simulink model "lidar_obstacle"  (R2020b)
settings: Solver=VariableStepAuto  StartTime=0.0  StopTime=Tf  RelTol=1e-3
values from neighbouring files (symbols this model uses):
  maze = imcomplement(maze)    [Run_Sim_LC.m]
  N = size(waypoints, 1)    [interpolate_leg_waypoints.m]
  startPose = [2 2 0]    [Run_Sim_LC.m]
  Ts = 0.01    [Run_Sim_LC.m]
  x = k4*t^4 + k3*t^3 + k2*t^2 + k1*t + k0    [get_leg_waypoints_symb.m]    (also in leg_ik_symb.m = r*cos(phi); leg_ik_symb_hexa.m = r*cos(phi+alpha))
  y = r*sin(phi)    [leg_ik_symb.m]    (also in leg_ik_symb_hexa.m = r*sin(phi+alpha))
undefined symbols (not defined in the file or in its folder): dimx, dimy, Discrete, mazeRes, thickness, Time, X, Y, Z
libraries: sm_lib x92, nesl_utility x4, robotics_pg_exp_pack x3, hexapod x2, RoboticsPlayground x1, ctrlSharedLib x1
settings Model: Creator=fciriell  LastModifiedBy=Leone
settings ExplorerConfigSet: InternalSimMechanicsExplorerSettings="<ExplorerConfiguration><canonicalview>default</canonicalview><AnimationSetting><BasePlaybackSpeed>1.0</BasePlaybackSpeed><PlaybackSpeedFactor>1.0</PlaybackSpeedFactor></AnimationSetting><TilePanel><TileInfo><Tiles Columns=\"1\" Count=\"2\" Rows=\"2\"><Column Weight=\"1\"/><Row Weight=\"0.4993\"/><Row Weight=\"0.5007\"/><Tile Height=\"1\" Width=\"1\" X=\"0\" Y=\"0\"/><Tile Height=\"1\" Width=\"1\" X=\"0\" Y=\"1\"/></Tiles></TileInfo><SceneInfo><SceneViewer><BGColor><R>1</R><G>1</G><B>1</B></BGColor><Camera><DoPerspective>on</DoPerspective><Position><X>-4.35147948962821829e-06</X><Y>-4.89869399804638128</Y><Z>0.176731420553238427</Z></Position><Center><X>-4.35147948962821829e-06</X><Y>-1.26250265135058726</Y><Z>0.176731420553238427</Z></Center><Up><X>0</X><Y>-0</Y><Z>1</Z></Up><ViewLimDist>1</ViewLimDist><YLim>0.466307658154998583</YLim><XLim>1.59125758717581123</XLim></Camera></SceneViewer><SceneViewer><BGColor><R>1</R><G>1</G><B>1</B></BGColor><Camera><DoPerspective>off</DoPerspective><Position><X>-5.9945065800093289e-08</X><Y>-3.21515629578642415</Y><Z>0.0606596897011122405</Z></Position><Center><X>-5.9945065800093289e-08</X><Y>-1.26250000733898382</Y><Z>0.0606596897011122405</Z></Center><Up><X>-0</X><Y>0</Y><Z>1</Z></Up><ViewLimDist>1</ViewLimDist><YLim>0.993270539045333911</YLim><XLim>3.37947076894122489</XLim></Camera></SceneViewer></SceneInfo></TilePanel><MechEditorPanel><Cameras><Camera><Id>Camera1</Id><Value><Name>Camera1</Name><NativeCamera><PositionTrackingFeature>camera.F</PositionTrackingFeature><CenterTrackingFeature>One_link_chain_dynamic.to_WF</CenterTrackingFeature><UpVectorTrackingFeature>camera.F</UpVectorTrackingFeature><CenterTrackingOrigin>on</CenterTrackingOrigin><UpVectorTrackingDirection>+Z</UpVectorTrackingDirection></NativeCamera></Value></Camera></Cameras><GfxPanelCameraMap><MapElement CameraMLId=\"Camera1\" GfxPanelIndex=\"0\"/></GfxPanelCameraMap><VideoCreator><PlaybackSpeedRatio>1.0</PlaybackSpeedRatio><FrameRate>30</FrameRate><VideoFormat>Motion JPEG AVI</VideoFormat><FrameSize>auto</FrameSize></VideoCreator></MechEditorPanel></ExplorerConfiguration>"

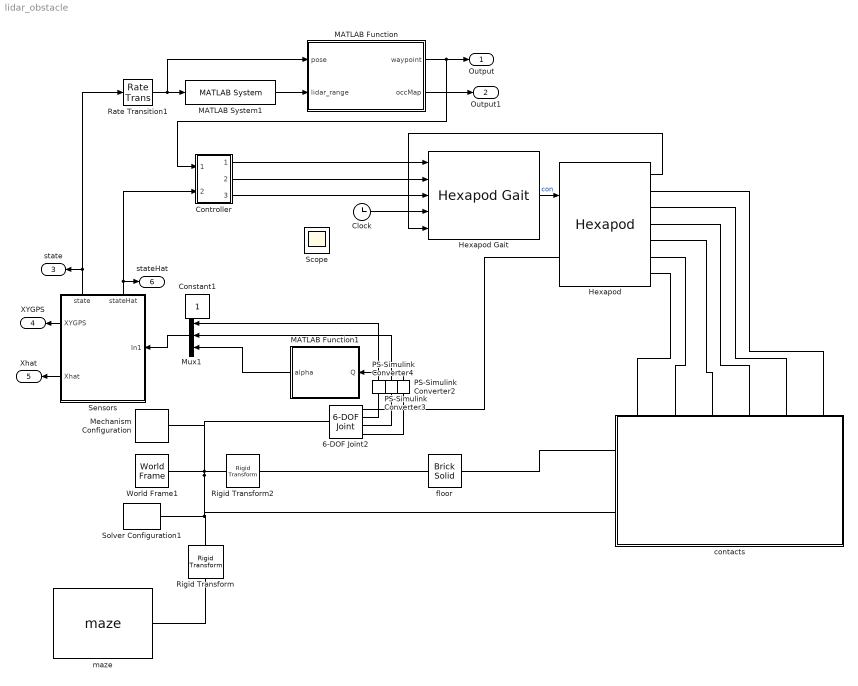
== system lidar_obstacle ==
  6-DOF Joint2 : sm_lib/Joints/6-DOF Joint  JointMode=Normal  SenseConstraintForce=off  SenseConstraintForceX=off  SenseConstraintForceY=off  SenseConstraintForceZ=off  SenseConstraintTorque=off  SenseConstraintTorqueX=off  SenseConstraintTorqueY=off  SenseConstraintTorqueZ=off  SenseTotalForce=off  SenseTotalForceX=off  SenseTotalForceY=off  SenseTotalForceZ=off  SenseTotalTorque=off  SenseTotalTorqueX=off  SenseTotalTorqueY=off  SenseTotalTorqueZ=off  CompositeWrenchDir=FollowerOnBase  CompositeWrenchFrame=BaseFrame  PxEquilibriumPosition=0  PxEquilibriumPositionUnits=m  PxSpringStiffness=0  PxSpringStiffnessUnits=N/m  PxDampingCoefficient=0  PxDampingCoefficientUnits=N/(m/s)  PxTorqueActuationMode=NoTorque  PxMotionActuationMode=ComputedMotion  PxSensePosition=on  PxSenseVelocity=off  PxSenseAcceleration=off  PxSenseTorqueForce=off  PxSenseLowerLimitTorqueForce=off  PxSenseUpperLimitTorqueForce=off  PxLowerLimitSpecify=off  PxLowerLimitBound=-1  PxLowerLimitBoundUnits=m  PxLowerLimitStiffness=1e6  PxLowerLimitStiffnessUnits=N/m  PxLowerLimitDamping=1e3  PxLowerLimitDampingUnits=N/(m/s)  PxLowerLimitTransitionRegionWidth=1e-4  PxLowerLimitTransitionRegionWidthUnits=m  PxUpperLimitSpecify=off  PxUpperLimitBound=1  PxUpperLimitBoundUnits=m  PxUpperLimitStiffness=1e6  PxUpperLimitStiffnessUnits=N/m  PxUpperLimitDamping=1e3  PxUpperLimitDampingUnits=N/(m/s)  PxUpperLimitTransitionRegionWidth=1e-4  PxUpperLimitTransitionRegionWidthUnits=m  PxPositionTargetSpecify=on  PxPositionTargetPriority=High  PxPositionTargetValue=startPose(1)  PxPositionTargetValueUnits=m  PxVelocityTargetSpecify=off  PxVelocityTargetPriority=High  PxVelocityTargetValue=0  PxVelocityTargetValueUnits=m/s  PyEquilibriumPosition=0  PyEquilibriumPositionUnits=m  PySpringStiffness=0  PySpringStiffnessUnits=N/m  PyDampingCoefficient=0  PyDampingCoefficientUnits=N/(m/s)  PyTorqueActuationMode=NoTorque  PyMotionActuationMode=ComputedMotion  PySensePosition=on  PySenseVelocity=off  PySenseAcceleration=off  PySenseTorqueForce=off  PySenseLowerLimitTorqueForce=off  PySenseUpperLimitTorqueForce=off  PyLowerLimitSpecify=off  PyLowerLimitBound=-1  PyLowerLimitBoundUnits=m  PyLowerLimitStiffness=1e6  PyLowerLimitStiffnessUnits=N/m  PyLowerLimitDamping=1e3  PyLowerLimitDampingUnits=N/(m/s)  PyLowerLimitTransitionRegionWidth=1e-4  PyLowerLimitTransitionRegionWidthUnits=m  PyUpperLimitSpecify=off  PyUpperLimitBound=1  PyUpperLimitBoundUnits=m  PyUpperLimitStiffness=1e6  PyUpperLimitStiffnessUnits=N/m  PyUpperLimitDamping=1e3  PyUpperLimitDampingUnits=N/(m/s)  PyUpperLimitTransitionRegionWidth=1e-4  PyUpperLimitTransitionRegionWidthUnits=m  PyPositionTargetSpecify=on  PyPositionTargetPriority=High  PyPositionTargetValue=startPose(2)  PyPositionTargetValueUnits=m  PyVelocityTargetSpecify=off  PyVelocityTargetPriority=High  PyVelocityTargetValue=0  PyVelocityTargetValueUnits=m/s  PzEquilibriumPosition=0  PzEquilibriumPositionUnits=m  PzSpringStiffness=0  PzSpringStiffnessUnits=N/m  PzDampingCoefficient=0  PzDampingCoefficientUnits=N/(m/s)  PzTorqueActuationMode=NoTorque  PzMotionActuationMode=ComputedMotion  PzSensePosition=off  PzSenseVelocity=off  PzSenseAcceleration=off  PzSenseTorqueForce=off  PzSenseLowerLimitTorqueForce=off  PzSenseUpperLimitTorqueForce=off  PzLowerLimitSpecify=off  PzLowerLimitBound=-1  PzLowerLimitBoundUnits=m  PzLowerLimitStiffness=1e6  PzLowerLimitStiffnessUnits=N/m  PzLowerLimitDamping=1e3  PzLowerLimitDampingUnits=N/(m/s)  PzLowerLimitTransitionRegionWidth=1e-4  PzLowerLimitTransitionRegionWidthUnits=m  PzUpperLimitSpecify=off  PzUpperLimitBound=1  PzUpperLimitBoundUnits=m  PzUpperLimitStiffness=1e6  PzUpperLimitStiffnessUnits=N/m  PzUpperLimitDamping=1e3  PzUpperLimitDampingUnits=N/(m/s)  PzUpperLimitTransitionRegionWidth=1e-4  PzUpperLimitTransitionRegionWidthUnits=m  PzPositionTargetSpecify=on  PzPositionTargetPriority=High  PzPositionTargetValue=0.35  PzPositionTargetValueUnits=m  PzVelocityTargetSpecify=off  PzVelocityTargetPriority=High  PzVelocityTargetValue=0  PzVelocityTargetValueUnits=m/s  SphDefPosRotationMethod=None  SphDefPosRotationAngleUnits=deg  SphDefPosRotationStandardAxis=+Z  SphDefPosRotationAngle=0.0  SphDefPosRotationArbitraryAxis=[0 0 1]  SphDefPosFollAlignAxisA=+X  SphDefPosBaseAlignAxisA=+Y  SphDefPosFollAlignAxisB=+Y  SphDefPosBaseAlignAxisB=+Z  SphDefPosRotationSequenceAxes=FollowerAxes  SphDefPosRotationSequence=XYX  SphDefPosRotationSequenceAngles=[0 0 0]  SphDefPosRotationSequenceAnglesUnits=deg  SphDefPosRotationMatrix=[1 0 0; 0 1 0; 0 0 1]  SphEqPosRotationMethod=None  SphEqPosRotationAngleUnits=deg  SphEqPosRotationStandardAxis=+Z  SphEqPosRotationAngle=0.0  SphEqPosRotationArbitraryAxis=[0 0 1]  SphEqPosFollAlignAxisA=+X  SphEqPosBaseAlignAxisA=+Y  SphEqPosFollAlignAxisB=+Y  SphEqPosBaseAlignAxisB=+Z  SphEqPosRotationSequenceAxes=FollowerAxes  SphEqPosRotationSequence=XYX  SphEqPosRotationSequenceAngles=[0 0 0]  SphEqPosRotationSequenceAnglesUnits=deg  SphEqPosRotationMatrix=[1 0 0; 0 1 0; 0 0 1]  SphSpringStiffness=0  SphSpringStiffnessUnits=N*m/deg  SphDampingCoefficient=0  SphDampingCoefficientUnits=N*m/(deg/s)  SphActuateTorqueX=off  SphActuateTorqueY=off  SphActuateTorqueZ=off  SphActuateTorque=off  SphTorqueActuationMode=NoTorque  SphMotionActuationMode=ComputedMotion  SphActuationFrame=BaseFrame  SphSensePosition=on  SphSenseVelocityX=off  SphSenseVelocityY=off  SphSenseVelocityZ=off  SphSenseVelocity=off  SphSenseAccelerationX=off  SphSenseAccelerationY=off  SphSenseAccelerationZ=off  SphSenseAcceleration=off  SphSenseTorqueX=off  SphSenseTorqueY=off  SphSenseTorqueZ=off  SphSenseTorqueForce=off  SphSenseLowerLimitTorqueMag=off  SphSenseUpperLimitTorqueMag=off  SphSensingFrame=BaseFrame  SphLowerLimitSpecify=off  SphLowerLimitBound=15  SphLowerLimitBoundUnits=deg  SphLowerLimitStiffness=1e4  SphLowerLimitStiffnessUnits=N*m/deg  SphLowerLimitDamping=10  SphLowerLimitDampingUnits=N*m/(deg/s)  SphLowerLimitTransitionRegionWidth=0.1  SphLowerLimitTransitionRegionWidthUnits=deg  SphUpperLimitSpecify=off  SphUpperLimitBound=45  SphUpperLimitBoundUnits=deg  SphUpperLimitStiffness=1e4  SphUpperLimitStiffnessUnits=N*m/deg  SphUpperLimitDamping=10  SphUpperLimitDampingUnits=N*m/(deg/s)  SphUpperLimitTransitionRegionWidth=0.1  SphUpperLimitTransitionRegionWidthUnits=deg  SphPositionTargetRotationMethod=None  SphPositionTargetRotationAngleUnits=deg  SphPositionTargetRotationStandardAxis=+Z  SphPositionTargetRotationAngle=0.0  SphPositionTargetRotationArbitraryAxis=[0 0 1]  SphPositionTargetFollAlignAxisA=+X  SphPositionTargetBaseAlignAxisA=+Y  SphPositionTargetFollAlignAxisB=+Y  SphPositionTargetBaseAlignAxisB=+Z  SphPositionTargetRotationSequenceAxes=FollowerAxes  SphPositionTargetRotationSequence=XYX  SphPositionTargetRotationSequenceAngles=[0 0 0]  SphPositionTargetRotationSequenceAnglesUnits=deg  SphPositionTargetRotationMatrix=[1 0 0; 0 1 0; 0 0 1]  SphPositionTargetSpecify=off  SphPositionTargetPriority=High  SphVelocityTargetValue=[0 0 0]  SphVelocityTargetValueUnits=deg/s  SphVelocityTargetSpecify=off  SphVelocityTargetPriority=High  SphVelocityTargetInFollowerFrame=on
  Clock : Clock
  Controller : Subsystem
  Hexapod : hexapod/Hexapod  leg_initial_config=[0; -pi/8; 5*pi/8]  leg_length_1=0.1  leg_length_2=0.4  leg_length_3=0.4  leg_radius=0.04  leg_mass_1=0.1  leg_mass_2=0.3  leg_mass_3=0.3  pos_kp=[80; 80; 80]  pos_ki=[0; 0; 0]  pos_kd=[10; 10; 10]  body_radius=0.3  body_mass=0.2
      settings: SourceProductName=Hexapod
  Hexapod Gait : hexapod/Hexapod Gait  beta=0.55  T=0.5  contact_start_config=[0; -pi/8; 5*pi/8]  lifted_mid_theta2=-pi/4  lifted_mid_theta3=3*pi/4  body_radius=0.3  leg_length_1=0.1  leg_length_2=0.4  leg_length_3=0.4
      settings: SourceProductName=Hexapod
  MATLAB Function : MATLAB Function  TreatAsAtomicUnit=on
  MATLAB Function1 : MATLAB Function  TreatAsAtomicUnit=on
  MATLAB System1 : RoboticsPlayground/Advanced Sensors/360 Range Sensor/MATLAB System  mapName=map  sensorOffset=[0 0]  scanAngles=linspace(-pi, pi, 50)  maxRange=6
      settings: SourceProductName=Robotics Playground
  Mechanism Configuration : sm_lib/Utilities/Mechanism Configuration  UniformGravity=Constant  GravityVector=[0 0 -9.80665]  GravityVectorUnits=m/s^2  GravityUnits=m/s^2  LinearizationDelta=0.001  JointModeTransitionNonlinearIterations=2
  Mux1 : Mux  Inputs=3
  PS-Simulink Converter2 : nesl_utility/PS-Simulink Converter  PhysicalDomain=network_engine_domain  SubClassName=ps_output  LeftPortType=input  RightPortType=output  PseudoPeriodic=off  Frequencies=[]  Unit=inherit  AffineConversion=off
  PS-Simulink Converter3 : nesl_utility/PS-Simulink Converter  PhysicalDomain=network_engine_domain  SubClassName=ps_output  LeftPortType=input  RightPortType=output  PseudoPeriodic=off  Frequencies=[]  Unit=inherit  AffineConversion=off
  PS-Simulink Converter4 : nesl_utility/PS-Simulink Converter  PhysicalDomain=network_engine_domain  SubClassName=ps_output  LeftPortType=input  RightPortType=output  PseudoPeriodic=off  Frequencies=[]  Unit=inherit  AffineConversion=off
  Rate Transition1 : RateTransition  OutPortSampleTime=Ts*5
  Rigid Transform : sm_lib/Frames and Transforms/Rigid Transform  TranslationMethod=StandardAxis  TranslationStandardOffset=0.255  TranslationLengthUnit=m  TranslationStandardAxis=-Z  TranslationCartesianOffset=[0 0 0]  TranslationROffset=0  TranslationROffsetUnits=m  TranslationZOffset=0  TranslationZOffsetUnits=m  TranslationThetaOffset=0  TranslationThetaOffsetUnits=deg  RotationMethod=None  RotationAngleUnits=deg  RotationStandardAxis=+Z  RotationAngle=0.0  RotationArbitraryAxis=[0 0 1]  FollAlignAxisA=+X  BaseAlignAxisA=+Y  FollAlignAxisB=+Y  BaseAlignAxisB=+Z  RotationSequenceAxes=FollowerAxes  RotationSequence=XYX  RotationSequenceAngles=[0 0 0]  RotationSequenceAnglesUnits=deg  RotationMatrix=[1 0 0; 0 1 0; 0 0 1]
  Rigid Transform2 : sm_lib/Frames and Transforms/Rigid Transform  TranslationMethod=Cartesian  TranslationStandardOffset=0  TranslationLengthUnit=m  TranslationStandardAxis=+Z  TranslationCartesianOffset=[0.5*size(maze, 2)/mazeRes 0.5*size(maze, 1)/mazeRes -0.25]  TranslationROffset=0  TranslationROffsetUnits=m  TranslationZOffset=0  TranslationZOffsetUnits=m  TranslationThetaOffset=0  TranslationThetaOffsetUnits=deg  RotationMethod=None  RotationAngleUnits=deg  RotationStandardAxis=+Z  RotationAngle=0.0  RotationArbitraryAxis=[0 0 1]  FollAlignAxisA=+X  BaseAlignAxisA=+Y  FollAlignAxisB=+Y  BaseAlignAxisB=+Z  RotationSequenceAxes=FollowerAxes  RotationSequence=XYX  RotationSequenceAngles=[0 0 0]  RotationSequenceAnglesUnits=deg  RotationMatrix=[1 0 0; 0 1 0; 0 0 1]
  Sensors : Subsystem
      settings: PortSchema="{\"entries\":[{\"content\":{\"sides\":[{\"content\":{\"connectorIds\":[\"In1\"]},\"type\":\"ConnectorPlacement.EquallySpacedRectSide\",\"uuid\":\"8db747f0-83c9-4cc5-b80c-4fdc53357bd0\"},{\"content\":{\"connectorIds\":[\"Out1\",\"Out2\"],\"side\":\"RIGHT\"},\"type\":\"ConnectorPlacement.EquallySpacedRectSide\",\"uuid\":\"410b3c6d-2c21-47e1-b07d-c9646b429a39\"},{\"content\":{\"connectorIds\":[\"Out3\",\"Out4\"],\"side\":\"TOP\"},\"type\":\"ConnectorPlacement.EquallySpacedRectSide\",\"uuid\":\"d7e8c555-6057-488c-b5e8-2079a1227ab0\"},{\"content\":{\"connectorIds\":[],\"side\":\"HIDDEN\"},\"type\":\"ConnectorPlacement.EquallySpacedRectSide\",\"uuid\":\"2e052cb0-9706-477d-91df-361bb344069c\"}]},\"type\":\"ConnectorPlacement.EquallySpacedConnector\",\"uuid\":\"19d42c93-4e78-4ee2-ba10-4e9242e82cdf\"}],\"packageUris\":[\"http://schema.mathworks.com/mf0/Connector/R2020b\"],\"version\":\"1.0\"}"
  Solver Configuration1 : nesl_utility/Solver Configuration  PhysicalDomain=network_engine_domain  SubClassName=solver  LeftPortType=input  RightPortType=generic  Tones=[]  Harmonics=[]  SimulateNoise=off  Profile=off  UseLocalSampling=off  EnableSwitchedLinearOptims=on  FrequencyDomain=off  UseCCode=off  RelTol=0.001  AbsTol=1e-06  MinStep=1e-09  ToWorkspace=off  RevertToSquareIcSolve=off  NumHomotopyIterations=100  PhasorMode=off  PhasorModeNumHarmonics=1  DoDC=off  ResidualTolerance=1e-09  UseLocalSolver=off  LocalSolverChoice=NE_BACKWARD_EULER_ADVANCER  LocalSolverSampleTime=0.001  DoFixedCost=off  MaxNonlinIter=3  MaxModeIter=2  ComputeImpulses=off  ImpulseIterations=2  LinearAlgebra=auto  EquationFormulation=NE_TIME_EF  DelaysMemoryBudget=1024  AutomaticFiltering=on  FilteringTimeConstant=0.001  PartitionStorageMethod=AS_NEEDED  PartitionMemoryBudget=1024  PartitionMethod=ROBUST
  World Frame1 : sm_lib/Frames and Transforms/World Frame
  contacts : Subsystem
      settings: PortSchema="{\"entries\":[{\"content\":{\"sides\":[{\"content\":{\"connectorIds\":[\"LConn1\",\"LConn2\"]},\"type\":\"ConnectorPlacement.EquallySpacedRectSide\",\"uuid\":\"cb8f013f-d070-4036-9a1e-b1da7f0524a2\"},{\"content\":{\"connectorIds\":[],\"side\":\"RIGHT\"},\"type\":\"ConnectorPlacement.EquallySpacedRectSide\",\"uuid\":\"90d98404-2ea8-4d7a-9f25-dfdb418498bc\"},{\"content\":{\"connectorIds\":[\"LConn3\",\"LConn4\",\"LConn5\",\"LConn6\",\"LConn7\",\"LConn8\"],\"side\":\"TOP\"},\"type\":\"ConnectorPlacement.EquallySpacedRectSide\",\"uuid\":\"f681a791-5d2e-4e59-97ef-d7602497293d\"},{\"content\":{\"connectorIds\":[],\"side\":\"HIDDEN\"},\"type\":\"ConnectorPlacement.EquallySpacedRectSide\",\"uuid\":\"413999c2-851c-41f9-9c6a-b2c6650b1a6d\"}]},\"type\":\"ConnectorPlacement.EquallySpacedConnector\",\"uuid\":\"d2e28969-11aa-474d-9e03-ac352d25b509\"}],\"packageUris\":[\"http://schema.mathworks.com/mf0/Connector/R2020b\"],\"version\":\"1.0\"}"
  floor : sm_lib/Body Elements/Brick Solid  GraphicAmbientColor=[0.15 0.15 0.15 1.0]  BasedOnType=Density  BrickDimensions=[size(maze, 1)/mazeRes size(maze, 2)/mazeRes 0.5]  BrickDimensionUnits=m  CenterOfMass=[0 0 0]  CenterOfMassUnits=m  GraphicDiffuseColor=[0.5 0.5 0.5]  Density=1000  DensityUnits=kg/m^3  DoExposeReferenceFrame=off  GraphicEmissiveColor=[0.0 0.0 0.0 1.0]  ExportEntireGeometry=on  SerializedFrames=<Frames><Frame><Id>Frame1</Id><Value><Name>TF</Name><Origin><Source>GeometricFeature</Source><FeatureName>+z surface</FeatureName></Origin><PrimaryAxis><DefinedDirection>+Z</DefinedDirection><Source>ReferenceFrame</Source><SourceDirection>+Z</SourceDirection><FeatureName></FeatureName></PrimaryAxis><SecondaryAxis><DefinedDirection>+X</DefinedDirection><Source>ReferenceFrame</Source><SourceDirection>+X</SourceDirection><FeatureName></FeatureName></SecondaryAxis></Value></Frame></Frames>  MarkerShape=Sphere  MarkerSize=10  GraphicType=FromGeometry  InertiaType=CalculateFromGeometry  Mass=1  MassUnits=kg  MomentsOfInertia=[1 1 1]  MomentsOfInertiaUnits=kg*m^2  GraphicOpacity=0.5  ProductsOfInertia=[0 0 0]  ProductsOfInertiaUnits=kg*m^2  GraphicShininess=75  GraphicSpecularColor=[0.5 0.5 0.5 1.0]  GraphicVisPropType=SimpleVisualProperties
  maze : robotics_pg_exp_pack/Environments & Sensors/Simscape Multibody Environments/maze  map=maze  wall_height=0.5  resolution=mazeRes  branching=branching
      settings: SourceProductName=Robotics Playground Expansion Pack
  Output : Outport
  Output1 : Outport  Port=2
  state : Outport  Port=3
  XYGPS : Outport  Port=4
  Xhat : Outport  Port=5
  stateHat : Outport  Port=6
  Constant1 : Constant  IOType=siggen
  Scope : Scope
  wires:
  Hexapod Gait/1 -> Hexapod/1  "con"
  Hexapod/1 -> Hexapod Gait/5
  Clock/1 -> Hexapod Gait/4
  MATLAB System1/1 -> MATLAB Function/2(lidar_range)
  Rate Transition1/1 -> MATLAB Function/1(pose), MATLAB System1/1
  MATLAB Function/1(waypoint) -> Controller/1(In1), Output/1
  MATLAB Function/2(occMap) -> Output1/1
  Sensors/1(XYGPS) -> XYGPS/1
  Sensors/2(Xhat) -> Xhat/1
  Sensors/4(state) -> state/1, Rate Transition1/1
  Sensors/3(stateHat) -> Controller/2(In2), stateHat/1
  Controller/1(Out1) -> Hexapod Gait/1
  Controller/2(Out2) -> Hexapod Gait/2
  Controller/3(Out3) -> Hexapod Gait/3
  PS-Simulink Converter2/1 -> MATLAB Function1/1(Q)
  PS-Simulink Converter4/1 -> Mux1/1
  PS-Simulink Converter3/1 -> Mux1/2
  MATLAB Function1/1(alpha) -> Mux1/3
  Mux1/1 -> Sensors/1(In1)
  connections:
  Rigid Transform2/RConn1 -- floor/LConn1
  Solver Configuration1/RConn1 -- contacts/LConn2 -- 6-DOF Joint2/LConn1 -- Mechanism Configuration/RConn1 -- Rigid Transform2/LConn1 -- World Frame1/RConn1 -- Rigid Transform/LConn1
  maze/RConn1 -- Rigid Transform/RConn1
  contacts/LConn8 -- Hexapod/RConn1
  contacts/LConn7 -- Hexapod/RConn2
  contacts/LConn6 -- Hexapod/RConn3
  contacts/LConn5 -- Hexapod/RConn4
  contacts/LConn4 -- Hexapod/RConn5
  contacts/LConn3 -- Hexapod/RConn6
  contacts/LConn1 -- floor/RConn1
  PS-Simulink Converter4/LConn1 -- 6-DOF Joint2/RConn2
  PS-Simulink Converter3/LConn1 -- 6-DOF Joint2/RConn3
  6-DOF Joint2/RConn4 -- PS-Simulink Converter2/LConn1
  6-DOF Joint2/RConn1 -- Hexapod/LConn1

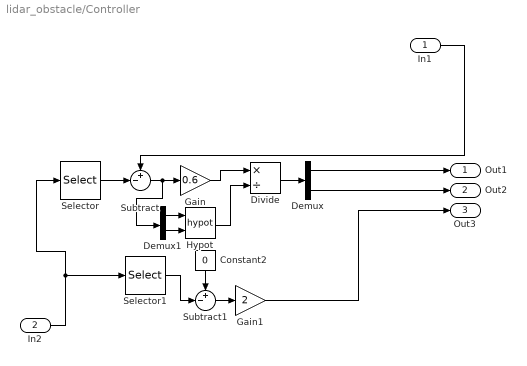
== system lidar_obstacle/Controller ==
  In1 : Inport
  In2 : Inport  Port=2
  Constant2 : Constant  Value=0
  Demux : Demux  Outputs=2
  Demux1 : Demux  Outputs=2
  Divide : Product  Inputs=*/
  Gain : Gain  Gain=0.6
  Gain1 : Gain  Gain=2
  Hypot : Math  Operator=hypot  SaturateOnIntegerOverflow=on
  Selector : Selector  InputPortWidth=3  IndexOptions=Index vector (dialog)  Indices=[1 2]  OutputSizes=1
  Selector1 : Selector  InputPortWidth=3  IndexOptions=Index vector (dialog)  Indices=[3]  OutputSizes=1
  Subtract : Sum  Inputs=+-|
  Subtract1 : Sum  Inputs=+-|
  Out1 : Outport
  Out2 : Outport  Port=2
  Out3 : Outport  Port=3
  wires:
  Hypot/1 -> Divide/2
  Subtract/1 -> Demux1/1, Gain/1
  Subtract1/1 -> Gain1/1
  Selector1/1 -> Subtract1/2
  In2/1 -> Selector/1, Selector1/1
  Selector/1 -> Subtract/2
  Demux1/2 -> Hypot/2
  Demux1/1 -> Hypot/1
  Divide/1 -> Demux/1
  Gain1/1 -> Out3/1
  Gain/1 -> Divide/1
  Constant2/1 -> Subtract1/1
  In1/1 -> Subtract/1
  Demux/2 -> Out2/1
  Demux/1 -> Out1/1

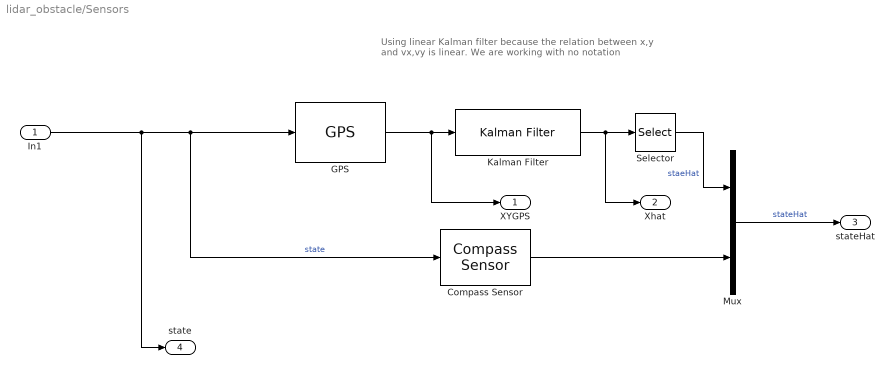
== system lidar_obstacle/Sensors ==
  note: Using linear Kalman filter because the relation between x,y and vx,vy is linear. We are working with no notation
  In1 : Inport
  "Compass Sensor " : robotics_pg_exp_pack/Environments & Sensors/Compass Sensor  sensorTs=0.1
      link override Rate Transition: InitialCondition=Ts
      settings: SourceProductName=Robotics Playground Expansion Pack
  "GPS " : robotics_pg_exp_pack/Environments & Sensors/GPS  xNoisePower=0.05  yNoisePower=0.05  Ts=Ts
      settings: SourceProductName=Robotics Playground Expansion Pack
  "Kalman Filter " : ctrlSharedLib/Kalman Filter  TimeDomain=Discrete-Time  UseCurrentEstimator=on  ModelSource=Individual A, B, C, D matrices  ModelSourceVariable=sys  A=[1 0 Ts 0; 0 1 0 Ts; 0 0 1 0; 0 0 0 1]  B=eye(2)  C=[1 0 0 0; 0 1 0 0]  D=zeros(2)  NumberOfStates=2  NumberOfInputs=2  NumberOfOutputs=2  InitialEstimateSource=Dialog  X0=0  P0=1e-3  UseK=off  UseGH=on  NumberOfProcessNoiseInputs=2  G=[Ts/2 0; 0 Ts/2; 1 0; 0 1]  TimeInvariantG=on  H=0  TimeInvariantH=on  Q=0.01  TimeInvariantQ=on  R=0.08  TimeInvariantR=on  N=0  TimeInvariantN=on  AddInputPort=off  AddEnablePort=off  OutputEstimatedY=off  OutputP=off  Ts=Ts
  Mux : Mux  Inputs=2
  Selector : Selector  InputPortWidth=4  IndexOptions=Index vector (dialog)  Indices=[1 2]  OutputSizes=1
  XYGPS : Outport
  Xhat : Outport  Port=2
  stateHat : Outport  Port=3
  state : Outport  Port=4
  wires:
  "GPS "/1 -> "Kalman Filter "/1, XYGPS/1
  "Kalman Filter "/1 -> Selector/1, Xhat/1
  "Compass Sensor "/1 -> Mux/2
  In1/1 -> state/1, "Compass Sensor "/1, "GPS "/1  "state"
  Mux/1 -> stateHat/1  "stateHat"
  Selector/1 -> Mux/1  "staeHat"

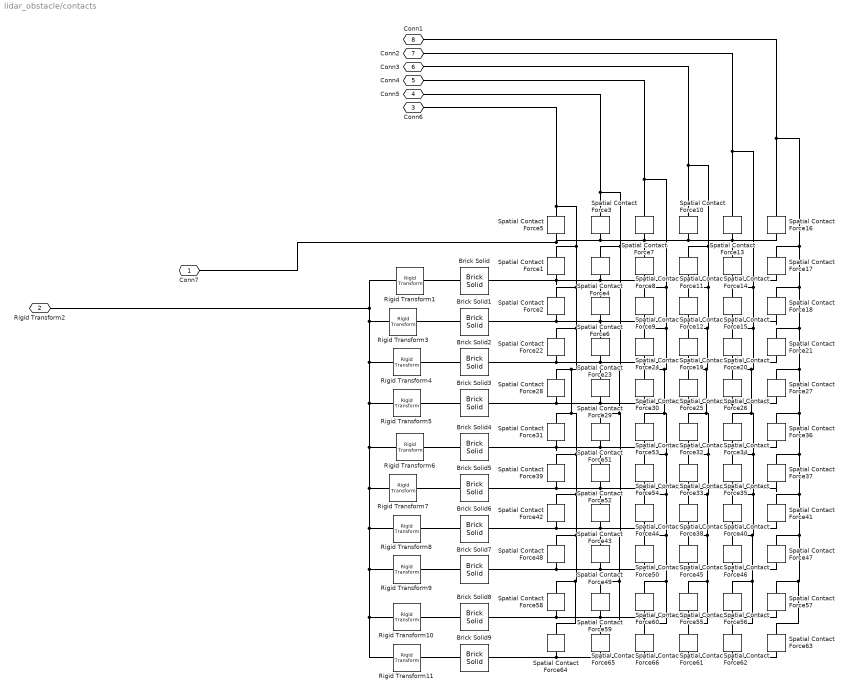
== system lidar_obstacle/contacts ==
  Brick Solid{,1..9} (10 alike) : sm_lib/Body Elements/Brick Solid  GraphicAmbientColor=[0.15 0.15 0.15 1.0]  BasedOnType=Density  BrickDimensions=[dimx dimy thickness]  BrickDimensionUnits=m  CenterOfMass=[0 0 0]  CenterOfMassUnits=m  GraphicDiffuseColor=[0.5 0.5 0.5]  Density=1000  DensityUnits=kg/m^3  DoExposeReferenceFrame=on  GraphicEmissiveColor=[0.0 0.0 0.0 1.0]  ExportEntireGeometry=on  SerializedFrames=<Frames/>  MarkerShape=Sphere  MarkerSize=10  GraphicType=FromGeometry  InertiaType=CalculateFromGeometry  Mass=1  MassUnits=kg  MomentsOfInertia=[1 1 1]  MomentsOfInertiaUnits=kg*m^2  GraphicOpacity=1.0  ProductsOfInertia=[0 0 0]  ProductsOfInertiaUnits=kg*m^2  GraphicShininess=75  GraphicSpecularColor=[0.5 0.5 0.5 1.0]  GraphicVisPropType=SimpleVisualProperties
  Rigid Transform1 : sm_lib/Frames and Transforms/Rigid Transform  TranslationMethod=Cartesian  TranslationStandardOffset=0  TranslationLengthUnit=m  TranslationStandardAxis=+Z  TranslationCartesianOffset=[x(1) y(1) -0.25]  TranslationROffset=0  TranslationROffsetUnits=m  TranslationZOffset=0  TranslationZOffsetUnits=m  TranslationThetaOffset=0  TranslationThetaOffsetUnits=deg  RotationMethod=None  RotationAngleUnits=deg  RotationStandardAxis=+Z  RotationAngle=0.0  RotationArbitraryAxis=[0 0 1]  FollAlignAxisA=+X  BaseAlignAxisA=+Y  FollAlignAxisB=+Y  BaseAlignAxisB=+Z  RotationSequenceAxes=FollowerAxes  RotationSequence=XYX  RotationSequenceAngles=[0 0 0]  RotationSequenceAnglesUnits=deg  RotationMatrix=[1 0 0; 0 1 0; 0 0 1]
  Rigid Transform10 : sm_lib/Frames and Transforms/Rigid Transform  TranslationMethod=Cartesian  TranslationStandardOffset=0  TranslationLengthUnit=m  TranslationStandardAxis=+Z  TranslationCartesianOffset=[x(9) y(9) -0.25]  TranslationROffset=0  TranslationROffsetUnits=m  TranslationZOffset=0  TranslationZOffsetUnits=m  TranslationThetaOffset=0  TranslationThetaOffsetUnits=deg  RotationMethod=None  RotationAngleUnits=deg  RotationStandardAxis=+Z  RotationAngle=0.0  RotationArbitraryAxis=[0 0 1]  FollAlignAxisA=+X  BaseAlignAxisA=+Y  FollAlignAxisB=+Y  BaseAlignAxisB=+Z  RotationSequenceAxes=FollowerAxes  RotationSequence=XYX  RotationSequenceAngles=[0 0 0]  RotationSequenceAnglesUnits=deg  RotationMatrix=[1 0 0; 0 1 0; 0 0 1]
  Rigid Transform11 : sm_lib/Frames and Transforms/Rigid Transform  TranslationMethod=Cartesian  TranslationStandardOffset=0  TranslationLengthUnit=m  TranslationStandardAxis=+Z  TranslationCartesianOffset=[x(10) y(10) -0.25]  TranslationROffset=0  TranslationROffsetUnits=m  TranslationZOffset=0  TranslationZOffsetUnits=m  TranslationThetaOffset=0  TranslationThetaOffsetUnits=deg  RotationMethod=None  RotationAngleUnits=deg  RotationStandardAxis=+Z  RotationAngle=0.0  RotationArbitraryAxis=[0 0 1]  FollAlignAxisA=+X  BaseAlignAxisA=+Y  FollAlignAxisB=+Y  BaseAlignAxisB=+Z  RotationSequenceAxes=FollowerAxes  RotationSequence=XYX  RotationSequenceAngles=[0 0 0]  RotationSequenceAnglesUnits=deg  RotationMatrix=[1 0 0; 0 1 0; 0 0 1]
  Rigid Transform3 : sm_lib/Frames and Transforms/Rigid Transform  TranslationMethod=Cartesian  TranslationStandardOffset=0  TranslationLengthUnit=m  TranslationStandardAxis=+Z  TranslationCartesianOffset=[x(2) y(2) -0.25]  TranslationROffset=0  TranslationROffsetUnits=m  TranslationZOffset=0  TranslationZOffsetUnits=m  TranslationThetaOffset=0  TranslationThetaOffsetUnits=deg  RotationMethod=None  RotationAngleUnits=deg  RotationStandardAxis=+Z  RotationAngle=0.0  RotationArbitraryAxis=[0 0 1]  FollAlignAxisA=+X  BaseAlignAxisA=+Y  FollAlignAxisB=+Y  BaseAlignAxisB=+Z  RotationSequenceAxes=FollowerAxes  RotationSequence=XYX  RotationSequenceAngles=[0 0 0]  RotationSequenceAnglesUnits=deg  RotationMatrix=[1 0 0; 0 1 0; 0 0 1]
  Rigid Transform4 : sm_lib/Frames and Transforms/Rigid Transform  TranslationMethod=Cartesian  TranslationStandardOffset=0  TranslationLengthUnit=m  TranslationStandardAxis=+Z  TranslationCartesianOffset=[x(3) y(3) -0.25]  TranslationROffset=0  TranslationROffsetUnits=m  TranslationZOffset=0  TranslationZOffsetUnits=m  TranslationThetaOffset=0  TranslationThetaOffsetUnits=deg  RotationMethod=None  RotationAngleUnits=deg  RotationStandardAxis=+Z  RotationAngle=0.0  RotationArbitraryAxis=[0 0 1]  FollAlignAxisA=+X  BaseAlignAxisA=+Y  FollAlignAxisB=+Y  BaseAlignAxisB=+Z  RotationSequenceAxes=FollowerAxes  RotationSequence=XYX  RotationSequenceAngles=[0 0 0]  RotationSequenceAnglesUnits=deg  RotationMatrix=[1 0 0; 0 1 0; 0 0 1]
  Rigid Transform5 : sm_lib/Frames and Transforms/Rigid Transform  TranslationMethod=Cartesian  TranslationStandardOffset=0  TranslationLengthUnit=m  TranslationStandardAxis=+Z  TranslationCartesianOffset=[x(4) y(4) -0.25]  TranslationROffset=0  TranslationROffsetUnits=m  TranslationZOffset=0  TranslationZOffsetUnits=m  TranslationThetaOffset=0  TranslationThetaOffsetUnits=deg  RotationMethod=None  RotationAngleUnits=deg  RotationStandardAxis=+Z  RotationAngle=0.0  RotationArbitraryAxis=[0 0 1]  FollAlignAxisA=+X  BaseAlignAxisA=+Y  FollAlignAxisB=+Y  BaseAlignAxisB=+Z  RotationSequenceAxes=FollowerAxes  RotationSequence=XYX  RotationSequenceAngles=[0 0 0]  RotationSequenceAnglesUnits=deg  RotationMatrix=[1 0 0; 0 1 0; 0 0 1]
  Rigid Transform6 : sm_lib/Frames and Transforms/Rigid Transform  TranslationMethod=Cartesian  TranslationStandardOffset=0  TranslationLengthUnit=m  TranslationStandardAxis=+Z  TranslationCartesianOffset=[x(5) y(5) -0.25]  TranslationROffset=0  TranslationROffsetUnits=m  TranslationZOffset=0  TranslationZOffsetUnits=m  TranslationThetaOffset=0  TranslationThetaOffsetUnits=deg  RotationMethod=None  RotationAngleUnits=deg  RotationStandardAxis=+Z  RotationAngle=0.0  RotationArbitraryAxis=[0 0 1]  FollAlignAxisA=+X  BaseAlignAxisA=+Y  FollAlignAxisB=+Y  BaseAlignAxisB=+Z  RotationSequenceAxes=FollowerAxes  RotationSequence=XYX  RotationSequenceAngles=[0 0 0]  RotationSequenceAnglesUnits=deg  RotationMatrix=[1 0 0; 0 1 0; 0 0 1]
  Rigid Transform7 : sm_lib/Frames and Transforms/Rigid Transform  TranslationMethod=Cartesian  TranslationStandardOffset=0  TranslationLengthUnit=m  TranslationStandardAxis=+Z  TranslationCartesianOffset=[x(6) y(6) -0.25]  TranslationROffset=0  TranslationROffsetUnits=m  TranslationZOffset=0  TranslationZOffsetUnits=m  TranslationThetaOffset=0  TranslationThetaOffsetUnits=deg  RotationMethod=None  RotationAngleUnits=deg  RotationStandardAxis=+Z  RotationAngle=0.0  RotationArbitraryAxis=[0 0 1]  FollAlignAxisA=+X  BaseAlignAxisA=+Y  FollAlignAxisB=+Y  BaseAlignAxisB=+Z  RotationSequenceAxes=FollowerAxes  RotationSequence=XYX  RotationSequenceAngles=[0 0 0]  RotationSequenceAnglesUnits=deg  RotationMatrix=[1 0 0; 0 1 0; 0 0 1]
  Rigid Transform8 : sm_lib/Frames and Transforms/Rigid Transform  TranslationMethod=Cartesian  TranslationStandardOffset=0  TranslationLengthUnit=m  TranslationStandardAxis=+Z  TranslationCartesianOffset=[x(7) y(7) -0.25]  TranslationROffset=0  TranslationROffsetUnits=m  TranslationZOffset=0  TranslationZOffsetUnits=m  TranslationThetaOffset=0  TranslationThetaOffsetUnits=deg  RotationMethod=None  RotationAngleUnits=deg  RotationStandardAxis=+Z  RotationAngle=0.0  RotationArbitraryAxis=[0 0 1]  FollAlignAxisA=+X  BaseAlignAxisA=+Y  FollAlignAxisB=+Y  BaseAlignAxisB=+Z  RotationSequenceAxes=FollowerAxes  RotationSequence=XYX  RotationSequenceAngles=[0 0 0]  RotationSequenceAnglesUnits=deg  RotationMatrix=[1 0 0; 0 1 0; 0 0 1]
  Rigid Transform9 : sm_lib/Frames and Transforms/Rigid Transform  TranslationMethod=Cartesian  TranslationStandardOffset=0  TranslationLengthUnit=m  TranslationStandardAxis=+Z  TranslationCartesianOffset=[x(8) y(8) -0.25]  TranslationROffset=0  TranslationROffsetUnits=m  TranslationZOffset=0  TranslationZOffsetUnits=m  TranslationThetaOffset=0  TranslationThetaOffsetUnits=deg  RotationMethod=None  RotationAngleUnits=deg  RotationStandardAxis=+Z  RotationAngle=0.0  RotationArbitraryAxis=[0 0 1]  FollAlignAxisA=+X  BaseAlignAxisA=+Y  FollAlignAxisB=+Y  BaseAlignAxisB=+Z  RotationSequenceAxes=FollowerAxes  RotationSequence=XYX  RotationSequenceAngles=[0 0 0]  RotationSequenceAnglesUnits=deg  RotationMatrix=[1 0 0; 0 1 0; 0 0 1]
  Spatial Contact Force{1,3..5,7..8,10..11,13..14,16..17,19..32,34,36,38,40..51,53,55..66} (54 alike) : sm_lib/Forces and Torques/Spatial Contact Force  CoefficientOfDynamicFriction=0.3  CoefficientOfStaticFriction=0.9  NormalDamping=1e3  NormalDampingUnits=N/(m/s)  NormalStiffness=1e6  NormalStiffnessUnits=N/m  FrictionalCriticalVelocity=1e-3  FrictionalCriticalVelocityUnits=m/s  ZeroCrossDetectContactStartAndEnd=off  SenseFrictionalForceMagnitude=off  SenseNormalForceMagnitude=off  SenseSeparationDistance=off  NormalTransitionRegionWidth=1e-4  NormalTransitionRegionWidthUnits=m  FrictionType=SmoothStickSlip
  Spatial Contact Force{2,6,9,12,15,18,33,35,37,39,52,54} (12 alike) : sm_lib/Forces and Torques/Spatial Contact Force  CoefficientOfDynamicFriction=1  CoefficientOfStaticFriction=1  NormalDamping=1e3  NormalDampingUnits=N/(m/s)  NormalStiffness=1e6  NormalStiffnessUnits=N/m  FrictionalCriticalVelocity=1e-3  FrictionalCriticalVelocityUnits=m/s  ZeroCrossDetectContactStartAndEnd=off  SenseFrictionalForceMagnitude=off  SenseNormalForceMagnitude=off  SenseSeparationDistance=off  NormalTransitionRegionWidth=1e-4  NormalTransitionRegionWidthUnits=m  FrictionType=SmoothStickSlip
  Conn7 : PMIOPort  Side=Left
  Rigid Transform2 : PMIOPort  Port=2  Side=Left
  Conn6 : PMIOPort  Port=3  Side=Left
  Conn5 : PMIOPort  Port=4  Side=Left
  Conn4 : PMIOPort  Port=5  Side=Left
  Conn3 : PMIOPort  Port=6  Side=Left
  Conn2 : PMIOPort  Port=7  Side=Left
  Conn1 : PMIOPort  Port=8  Side=Left
  connections:
  Spatial Contact Force52/RConn1 -- Spatial Contact Force29/RConn1 -- Spatial Contact Force23/RConn1 -- Conn5/RConn1 -- Spatial Contact Force3/RConn1 -- Spatial Contact Force4/RConn1 -- Spatial Contact Force6/RConn1 -- Spatial Contact Force51/RConn1 -- Spatial Contact Force65/RConn1 -- Spatial Contact Force59/RConn1 -- Spatial Contact Force49/RConn1 -- Spatial Contact Force43/RConn1
  Rigid Transform11/RConn1 -- Brick Solid9/RConn1
  Spatial Contact Force46/LConn1 -- Spatial Contact Force49/LConn1 -- Brick Solid7/LConn1 -- Spatial Contact Force48/LConn1 -- Spatial Contact Force50/LConn1 -- Spatial Contact Force45/LConn1 -- Spatial Contact Force47/LConn1
  Rigid Transform10/RConn1 -- Brick Solid8/RConn1
  Rigid Transform4/LConn1 -- Rigid Transform2/RConn1 -- Rigid Transform1/LConn1 -- Rigid Transform3/LConn1 -- Rigid Transform5/LConn1 -- Rigid Transform7/LConn1 -- Rigid Transform11/LConn1 -- Rigid Transform10/LConn1 -- Rigid Transform9/LConn1 -- Rigid Transform8/LConn1 -- Rigid Transform6/LConn1
  Rigid Transform1/RConn1 -- Brick Solid/RConn1
  Spatial Contact Force31/LConn1 -- Brick Solid4/LConn1 -- Spatial Contact Force51/LConn1 -- Spatial Contact Force53/LConn1 -- Spatial Contact Force36/LConn1 -- Spatial Contact Force34/LConn1 -- Spatial Contact Force32/LConn1
  Spatial Contact Force40/RConn1 -- Spatial Contact Force62/RConn1 -- Spatial Contact Force56/RConn1 -- Spatial Contact Force46/RConn1 -- Spatial Contact Force35/RConn1 -- Spatial Contact Force26/RConn1 -- Spatial Contact Force20/RConn1 -- Conn2/RConn1 -- Spatial Contact Force13/RConn1 -- Spatial Contact Force14/RConn1 -- Spatial Contact Force15/RConn1 -- Spatial Contact Force34/RConn1
  Spatial Contact Force41/RConn1 -- Spatial Contact Force63/RConn1 -- Spatial Contact Force57/RConn1 -- Spatial Contact Force47/RConn1 -- Spatial Contact Force37/RConn1 -- Conn1/RConn1 -- Spatial Contact Force16/RConn1 -- Spatial Contact Force17/RConn1 -- Spatial Contact Force18/RConn1 -- Spatial Contact Force21/RConn1 -- Spatial Contact Force27/RConn1 -- Spatial Contact Force36/RConn1
  Spatial Contact Force62/LConn1 -- Spatial Contact Force63/LConn1 -- Spatial Contact Force65/LConn1 -- Brick Solid9/LConn1 -- Spatial Contact Force64/LConn1 -- Spatial Contact Force66/LConn1 -- Spatial Contact Force61/LConn1
  Spatial Contact Force44/RConn1 -- Spatial Contact Force66/RConn1 -- Spatial Contact Force60/RConn1 -- Spatial Contact Force50/RConn1 -- Spatial Contact Force30/RConn1 -- Spatial Contact Force24/RConn1 -- Conn4/RConn1 -- Spatial Contact Force7/RConn1 -- Spatial Contact Force8/RConn1 -- Spatial Contact Force9/RConn1 -- Spatial Contact Force53/RConn1 -- Spatial Contact Force54/RConn1
  Spatial Contact Force32/RConn1 -- Spatial Contact Force33/RConn1 -- Spatial Contact Force61/RConn1 -- Spatial Contact Force55/RConn1 -- Spatial Contact Force45/RConn1 -- Spatial Contact Force38/RConn1 -- Spatial Contact Force25/RConn1 -- Spatial Contact Force19/RConn1 -- Spatial Contact Force12/RConn1 -- Spatial Contact Force11/RConn1 -- Conn3/RConn1 -- Spatial Contact Force10/RConn1
  Spatial Contact Force35/LConn1 -- Spatial Contact Force37/LConn1 -- Spatial Contact Force33/LConn1 -- Brick Solid5/LConn1 -- Spatial Contact Force39/LConn1 -- Spatial Contact Force52/LConn1 -- Spatial Contact Force54/LConn1
  Spatial Contact Force24/LConn1 -- Spatial Contact Force21/LConn1 -- Spatial Contact Force20/LConn1 -- Spatial Contact Force19/LConn1 -- Spatial Contact Force23/LConn1 -- Brick Solid2/LConn1 -- Spatial Contact Force22/LConn1
  Spatial Contact Force26/LConn1 -- Spatial Contact Force29/LConn1 -- Brick Solid3/LConn1 -- Spatial Contact Force28/LConn1 -- Spatial Contact Force30/LConn1 -- Spatial Contact Force25/LConn1 -- Spatial Contact Force27/LConn1
  Spatial Contact Force15/LConn1 -- Spatial Contact Force18/LConn1 -- Brick Solid1/LConn1 -- Spatial Contact Force2/LConn1 -- Spatial Contact Force6/LConn1 -- Spatial Contact Force9/LConn1 -- Spatial Contact Force12/LConn1
  Rigid Transform9/RConn1 -- Brick Solid7/RConn1
  Spatial Contact Force42/RConn1 -- Spatial Contact Force28/RConn1 -- Conn6/RConn1 -- Spatial Contact Force5/RConn1 -- Spatial Contact Force1/RConn1 -- Spatial Contact Force2/RConn1 -- Spatial Contact Force22/RConn1 -- Spatial Contact Force31/RConn1 -- Spatial Contact Force39/RConn1 -- Spatial Contact Force64/RConn1 -- Spatial Contact Force58/RConn1 -- Spatial Contact Force48/RConn1
  Rigid Transform7/RConn1 -- Brick Solid5/RConn1
  Rigid Transform8/RConn1 -- Brick Solid6/RConn1
  Rigid Transform6/RConn1 -- Brick Solid4/RConn1
  Rigid Transform3/RConn1 -- Brick Solid1/RConn1
  Spatial Contact Force60/LConn1 -- Spatial Contact Force57/LConn1 -- Spatial Contact Force56/LConn1 -- Spatial Contact Force55/LConn1 -- Spatial Contact Force59/LConn1 -- Brick Solid8/LConn1 -- Spatial Contact Force58/LConn1
  Spatial Contact Force1/LConn1 -- Brick Solid/LConn1 -- Spatial Contact Force17/LConn1 -- Spatial Contact Force14/LConn1 -- Spatial Contact Force11/LConn1 -- Spatial Contact Force8/LConn1 -- Spatial Contact Force4/LConn1
  Spatial Contact Force5/LConn1 -- Conn7/RConn1 -- Spatial Contact Force16/LConn1 -- Spatial Contact Force13/LConn1 -- Spatial Contact Force10/LConn1 -- Spatial Contact Force7/LConn1 -- Spatial Contact Force3/LConn1
  Rigid Transform4/RConn1 -- Brick Solid2/RConn1
  Rigid Transform5/RConn1 -- Brick Solid3/RConn1
  Spatial Contact Force44/LConn1 -- Spatial Contact Force41/LConn1 -- Spatial Contact Force40/LConn1 -- Spatial Contact Force38/LConn1 -- Spatial Contact Force43/LConn1 -- Brick Solid6/LConn1 -- Spatial Contact Force42/LConn1

== matlab function lidar_obstacle/MATLAB Function ==
  data: pose input; waypoint output; lidar_range input; occMap output
function [waypoint, occMap]= fcn(pose, lidar_range)
    startPose = [2 2 0];
    goalPose = [13 13 0];
    map_x_limits = [-2 20];
    map_y_limits = [-2 20];
    map_size = [148 149];
    map_res = 10;
    sensor_angles = linspace(-pi, pi, 50);
    max_range = 6;
    
    pose = [pose(1) pose(2) pose(3)];
    
    persistent ss map i current_waypoints waypoint_i;
    
    if isempty(ss)
        ss = stateSpaceSE2;
        ss.StateBounds = [map_x_limits; map_y_limits; -pi pi];
    end
    if isempty(map)
        base = zeros(map_size);
        base = imbinarize(base);
        map = binaryOccupancyMap(base, map_res);
    end
    if isempty(i)
        i = 1;
    end

    scan = lidarScan(lidar_range, sensor_angles);
    insertRay(map, pose, scan, max_range);

    if isempty(current_waypoints)
        validator = validatorOccupancyMap(ss);
        validator.Map = copy(map);
        validator.Map.inflate(1);
        planner = plannerRRTStar(ss, validator);
        planner.MaxIterations=1e6;
        planner.MaxNumTreeNodes=1e6;
        planner.MaxConnectionDistance = 0.4;
        [refpath, ~] = plan(planner, startPose, goalPose);
        current_waypoints = refpath.States(:,1:2);
        waypoint_i = 1;
    end
    
    i = i + 1;
    if i > 10
        i = 1;
        validator = validatorOccupancyMap(ss);
        validator.Map = copy(map);
        validator.Map.inflate(0.8);
        isValid = true;
        for j = waypoint_i:size(current_waypoints, 1)-1
            [thisValid, ~] = isMotionValid(...
                validator,...
                [current_waypoints(j,:) 0],...
                [current_waypoints(j+1,:) 0]...
            );
            if ~thisValid
                isValid = false;
                break;
            end
        end
        if ~isValid
            planner = plannerRRTStar(ss, validator);
            planner.MaxIterations=1e6;
            planner.MaxNumTreeNodes=1e6;
            planner.MaxConnectionDistance = 0.8;
            
            prevPose = [current_waypoints(waypoint_i,:) 0];
            [refpath, ~] = plan(planner, prevPose, goalPose);
            current_waypoints = refpath.States(:,1:2);
            waypoint_i = 1;
        end
    end
    
    waypoint = current_waypoints(waypoint_i, :);
    dist = hypot(pose(1)-waypoint(1), pose(2)-waypoint(2));
    if dist < 0.1 && waypoint_i < size(current_waypoints, 1)
        waypoint_i = waypoint_i + 1;
        waypoint = current_waypoints(waypoint_i, :);
    end
    occMap = zeros(148, 149);
    occMap2 = map.occupancyMatrix();
    occMap(1:148, 1:149) = occMap2(1:148, 1:149);
end

== matlab function lidar_obstacle/MATLAB Function1 ==
  data: Q input; alpha output
function alpha = angle(Q)
% Rotation matrix
R = [
    1-2*(Q(2)^2+Q(3)^2) 2*(Q(1)*Q(2)-Q(4)*Q(3)) 2*(Q(1)*Q(3)+Q(4)*Q(2));
    2*(Q(1)*Q(2)+Q(4)*Q(3)) 1-2*(Q(1)^2+Q(3)^2) 2*(Q(2)*Q(3)-Q(4)*Q(1));
    2*(Q(1)*Q(3)-Q(4)*Q(2)) 2*(Q(2)*Q(3)+Q(4)*Q(1)) 1-2*(Q(1)^2+Q(2)^2)
];
alpha = atan2(R(2,1), R(1,1));
end
